simulink model "FOSWEC"  (R2016a)
settings: Solver=ode4  StartTime=0  StopTime=15  FixedStep=0.01  RelTol=1e-3
undefined symbols (not defined in the file): body, constraint, mooring
libraries: WECSim_Lib x16
settings Model: Creator=cmichel  LastModifiedBy=kmruehl
settings DataIOCC: LimitDataPoints=on  SaveFormat=Array
settings DebuggingCC: SolverPrmCheckMsg=warning  AllowSymbolicDim=off
settings HardwareCC: ProdBitPerPointer=32  ProdLargestAtomicFloat=None  ProdIntDivRoundTo=Undefined  ProdEndianess=Unspecified  ProdWordSize=32  ProdHWDeviceType=32-bit Generic
settings ModelReferenceCC: PropagateSignalLabelsOutOfModel=off
settings ConfigComp: CovModelRefEnable=Off  CovSFcnEnable=off
settings ConfigurationSet: Description=SimMechanics 2G

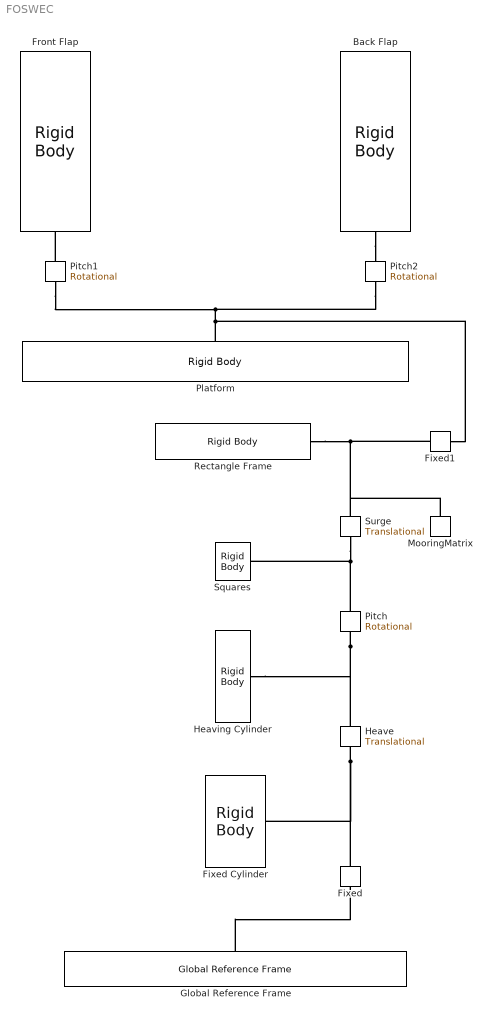
== system FOSWEC ==
  Back Flap : WECSim_Lib/Body Elements/Rigid Body  body=body(1)
      settings: AttributesFormatString=%<body>
  Fixed : WECSim_Lib/Constraints/Fixed  constraint=constraint(5)
      settings: AttributesFormatString=%<constraint>
  Fixed Cylinder : WECSim_Lib/Body Elements/Rigid Body  body=body(7)
      settings: AttributesFormatString=%<body>
  Fixed1 : WECSim_Lib/Constraints/Fixed  constraint=constraint(1)
      settings: AttributesFormatString=%<constraint>
  Front Flap : WECSim_Lib/Body Elements/Rigid Body  body=body(2)
      settings: AttributesFormatString=%<body>
  Global Reference Frame : WECSim_Lib/Frames/Global Reference Frame  waves=waves  simu=simu
  Heave : WECSim_Lib/Constraints/Translational  constraint=constraint(4)
      settings: AttributesFormatString=%<constraint>
  Heaving Cylinder : WECSim_Lib/Body Elements/Rigid Body  body=body(6)
      settings: AttributesFormatString=%<body>
  MooringMatrix : WECSim_Lib/Moorings/MooringMatrix  mooring=mooring(1)
      settings: AttributesFormatString=%<mooring>
  Pitch : WECSim_Lib/Constraints/Rotational  constraint=constraint(3)
      settings: AttributesFormatString=%<constraint>
  Pitch1 : WECSim_Lib/Constraints/Rotational  constraint=constraint(6)
      settings: AttributesFormatString=%<constraint>
  Pitch2 : WECSim_Lib/Constraints/Rotational  constraint=constraint(7)
      settings: AttributesFormatString=%<constraint>
  Platform : WECSim_Lib/Body Elements/Rigid Body  body=body(3)
      settings: AttributesFormatString=%<body>
  Rectangle Frame : WECSim_Lib/Body Elements/Rigid Body  body=body(4)
      settings: AttributesFormatString=%<body>
  Squares : WECSim_Lib/Body Elements/Rigid Body  body=body(5)
      settings: AttributesFormatString=%<body>
  Surge : WECSim_Lib/Constraints/Translational  constraint=constraint(2)
      settings: AttributesFormatString=%<constraint>
  connections:
  Back Flap/RConn1 -- Pitch2/RConn1
  Platform/RConn1 -- Fixed1/RConn1 -- Pitch2/LConn1 -- Pitch1/LConn1
  Global Reference Frame/RConn1 -- Fixed/LConn1
  Pitch/RConn1 -- Surge/LConn1 -- Squares/RConn1
  Rectangle Frame/RConn1 -- MooringMatrix/LConn1 -- Surge/RConn1 -- Fixed1/LConn1
  Pitch/LConn1 -- Heaving Cylinder/RConn1 -- Heave/RConn1
  Heave/LConn1 -- Fixed/RConn1 -- Fixed Cylinder/RConn1
  Pitch1/RConn1 -- Front Flap/RConn1
